simulink library "AccCellGroup"  (R2020a)
settings: Solver=VariableStepAuto  StartTime=0.0  StopTime=10.0  RelTol=1e-3
undefined symbols (not defined in the file or in its folder): DiscIntNeverNeededParam
libraries: simulink x2
settings Model: Creator=sean  LastModifiedBy=sean

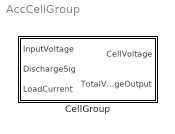
== system AccCellGroup ==
  CellGroup : Subsystem  mask{InitialSOCDefficit=18, InternalResistance=0.0018}
      mask prompts: InitialSOCDefficit "Initial SOC Deficit (Ah)"; InternalResistance "Internal Resistance (Ohms)"
      mask TypeOptions InitialSOCDefficit: SOCOffset/Value
      mask TypeOptions InternalResistance: InternalResistance/Value

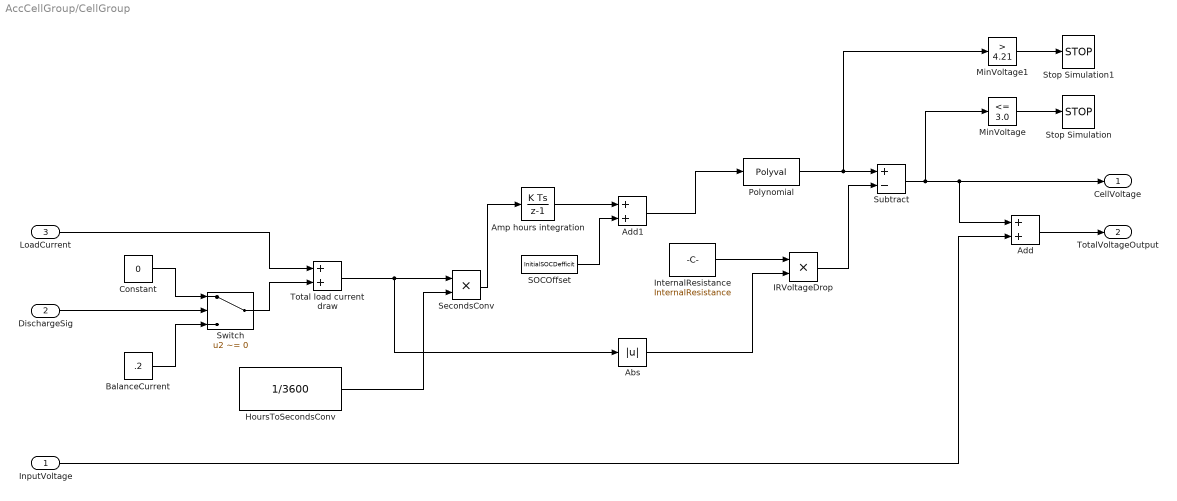
== system AccCellGroup/CellGroup ==
  InputVoltage : Inport
  DischargeSig : Inport  Port=2
  LoadCurrent : Inport  Port=3
  Abs : Abs
  Add : Sum
  Add1 : Sum
  Amp hours integration : DiscreteIntegrator  SampleTime=-1  ICPrevOutput=DiscIntNeverNeededParam  ICPrevScaledInput=DiscIntNeverNeededParam
  BalanceCurrent : Constant  Value=.2
  Constant : Constant  Value=0
  HoursToSecondsConv : Constant  Value=1/3600
  IRVoltageDrop : Product
  InternalResistance : Constant  Value=InternalResistance
  MinVoltage : simulink/Logic and Bit Operations/Compare To Constant  relop=<=  const=3.0  OutDataTypeStr=boolean
  MinVoltage1 : simulink/Logic and Bit Operations/Compare To Constant  relop=>  const=4.21  OutDataTypeStr=boolean
  Polynomial : Polyval  Coefs=[ -2.94E-4, 8.27E-3, -.0926, 4.2]
  SOCOffset : Constant  Value=InitialSOCDefficit
  SecondsConv : Product
  Stop Simulation : Stop
  Stop Simulation1 : Stop
  Subtract : Sum  Inputs=+-
  Switch : Switch  Criteria=u2 ~= 0
  Total load current draw : Sum
  CellVoltage : Outport
  TotalVoltageOutput : Outport  Port=2
  wires:
  DischargeSig/1 -> Switch/2
  BalanceCurrent/1 -> Switch/3
  Constant/1 -> Switch/1
  LoadCurrent/1 -> Total load current draw/1
  Switch/1 -> Total load current draw/2
  Total load current draw/1 -> Abs/1, SecondsConv/1
  SecondsConv/1 -> Amp hours integration/1
  HoursToSecondsConv/1 -> SecondsConv/2
  InternalResistance/1 -> IRVoltageDrop/1
  Polynomial/1 -> MinVoltage1/1, Subtract/1
  IRVoltageDrop/1 -> Subtract/2
  InputVoltage/1 -> Add/2
  Subtract/1 -> MinVoltage/1, Add/1, CellVoltage/1
  Add/1 -> TotalVoltageOutput/1
  Abs/1 -> IRVoltageDrop/2
  Amp hours integration/1 -> Add1/1
  Add1/1 -> Polynomial/1
  SOCOffset/1 -> Add1/2
  MinVoltage/1 -> Stop Simulation/1
  MinVoltage1/1 -> Stop Simulation1/1
